simulink library "INT_FlSys_FlConsTot"  (R2016b)
settings: Solver=VariableStepAuto  StartTime=0.0  StopTime=10.0  RelTol=1e-3
settings Model: Creator=yushengzhou  LastModifiedBy=yushengzhou

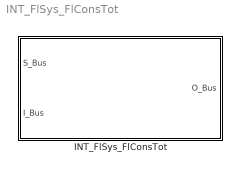
== system INT_FlSys_FlConsTot ==
  INT_FlSys_FlConsTot : Subsystem

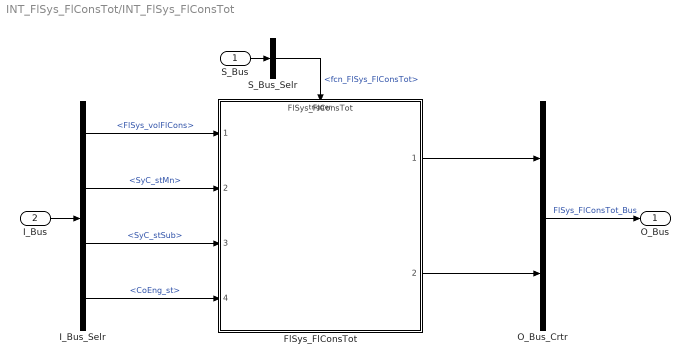
== system INT_FlSys_FlConsTot/INT_FlSys_FlConsTot ==
  S_Bus : Inport
  I_Bus : Inport  Port=2
  FlSys_FlConsTot : ModelReference  ModelNameDialog=FlSys_FlConsTot  SimulationMode=Normal  ModelReferenceVersion=1.14  TriggerPortName=function  TriggerPortTriggerType=function-call  TriggerPortStatesWhenEnabling=held
  I_Bus_Selr : BusSelector  OutputSignals=FlSys_volFlCons,SyC_stMn,SyC_stSub,CoEng_st
  O_Bus_Crtr : BusCreator  Inputs=2
  S_Bus_Selr : BusSelector  OutputSignals=fcn_FlSys_FlConsTot
  O_Bus : Outport
  wires:
  S_Bus_Selr/1 -> FlSys_FlConsTot/Trigger  "<fcn_FlSys_FlConsTot>"
  S_Bus/1 -> S_Bus_Selr/1
  I_Bus/1 -> I_Bus_Selr/1
  I_Bus_Selr/1 -> FlSys_FlConsTot/1  "<FlSys_volFlCons>"
  I_Bus_Selr/2 -> FlSys_FlConsTot/2  "<SyC_stMn>"
  I_Bus_Selr/3 -> FlSys_FlConsTot/3  "<SyC_stSub>"
  I_Bus_Selr/4 -> FlSys_FlConsTot/4  "<CoEng_st>"
  O_Bus_Crtr/1 -> O_Bus/1  "FlSys_FlConsTot_Bus"
  FlSys_FlConsTot/1 -> O_Bus_Crtr/1
  FlSys_FlConsTot/2 -> O_Bus_Crtr/2
